simulink model "Full_System_Test"  (R2023a)
settings: Solver=ode23tb  StartTime=0.0  StopTime=3  RelTol=1e-3
libraries: dspfdesign x8, dspsrcs4 x8, dspvision x2, dspxfrm3 x1
settings Model: Creator=zacha  LastModifiedBy=zacha
settings DebuggingCC: UnconnectedInputMsg=warning  UnconnectedOutputMsg=warning  UnconnectedLineMsg=warning
settings ModelReferenceCC: EnableRefExpFcnMdlSchedulingChecks=on
settings RTWCC: DLArmComputeVersion=19.05

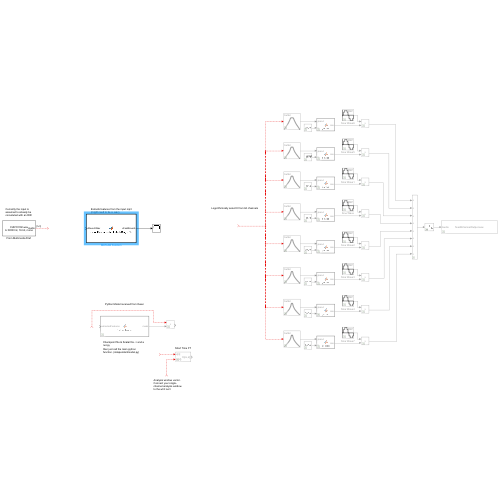
[thumbnail: Simulink's stored preview of the top-level diagram]
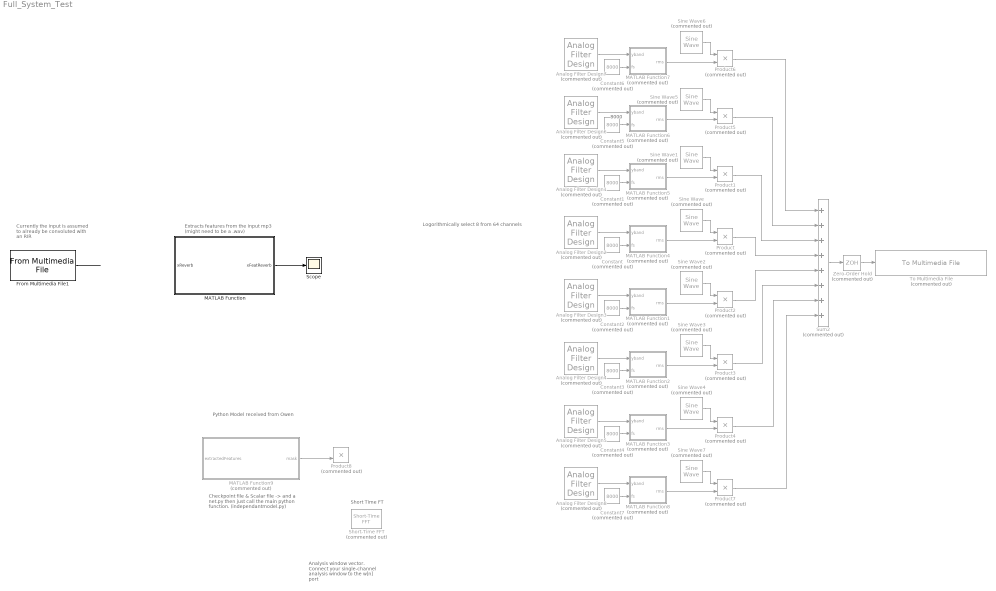
== system Full_System_Test ==
  note: Logorithmically select 8 from 64 channels
  note: Currently the input is assumed to already be convoluted with an RIR
  note: 8000
  note: Short Time FT
  note: Analysis window vector. Connect your single-channel analysis window to the w[n] port
  note: Checkpoint file & Scalar file -> and a net.py
      | then just call the main python function. (independantmodel.py)
  note: Python Model received from Owen
  note: Extracts features from the input mp3 (might need to be a .wav)
  Analog Filter Design1 : dspfdesign/Analog Filter Design  Commented=on  method=Butterworth  filttype=Bandpass  N=6  Wlo=5497.89355477605  Whi=8266.17682725960  Rp=2  Rs=40
  Analog Filter Design2 : dspfdesign/Analog Filter Design  Commented=on  method=Butterworth  filttype=Bandpass  N=6  Wlo=8266.17682725960  Whi=11762.6119981492  Rp=2  Rs=40
  Analog Filter Design3 : dspfdesign/Analog Filter Design  Commented=on  method=Butterworth  filttype=Bandpass  N=6  Wlo=11762.6119981492  Whi=16178.7275834830  Rp=2  Rs=40
  Analog Filter Design4 : dspfdesign/Analog Filter Design  Commented=on  method=Butterworth  filttype=Bandpass  N=6  Wlo=16178.7275834830  Whi=21756.4305609036  Rp=2  Rs=40
  Analog Filter Design5 : dspfdesign/Analog Filter Design  Commented=on  method=Butterworth  filttype=Bandpass  N=6  Wlo=21756.4305609036  Whi=28801.2576047532  Rp=2  Rs=40
  Analog Filter Design6 : dspfdesign/Analog Filter Design  Commented=on  method=Butterworth  filttype=Bandpass  N=6  Wlo=3306.12053392451  Whi=5497.89355477605  Rp=2  Rs=40
  Analog Filter Design7 : dspfdesign/Analog Filter Design  Commented=on  method=Butterworth  filttype=Bandpass  N=6  Wlo=1570.79632679490  Whi=3306.12053392451  Rp=2  Rs=40
  Analog Filter Design8 : dspfdesign/Analog Filter Design  Commented=on  method=Butterworth  filttype=Bandpass  N=6  Wlo=28801.2576047532  Whi=37699.1118430775  Rp=2  Rs=40
  Constant{,1..7} (8 alike) : Constant  Commented=on  Value=8000
  From Multimedia File1 : dspvision/From Multimedia File  inputFilename=C:\Users\zacha\Desktop\Cochlear\Media\zach reverb audio\zach reverb audio\CUNY0102.wav  readRange=[1 Inf]  loop=on  numPlays=1  outputStreams=Audio only  videoDataType=single  audioDataType=double  inheritSampleTime=off  userDefinedSampleTime=1/8000  noAudioOutput=off  isIntensityVideo=off  fourcc=RGB  colorVideoFormat=Separate color signals  outputEOF=off  dataOrg=Column-major  audioFrameSize=1  computeAudioFrameSize=off  outSamplingMode=Sample based
      settings: LibrarySourceBlock=dspsrcs4/From Multimedia File
  MATLAB Function : MATLAB Function  TreatAsAtomicUnit=on
  MATLAB Function1 : MATLAB Function  Commented=on  TreatAsAtomicUnit=on
  MATLAB Function2 : MATLAB Function  Commented=on  TreatAsAtomicUnit=on
  MATLAB Function3 : MATLAB Function  Commented=on  TreatAsAtomicUnit=on
  MATLAB Function4 : MATLAB Function  Commented=on  TreatAsAtomicUnit=on
  MATLAB Function5 : MATLAB Function  Commented=on  TreatAsAtomicUnit=on
  MATLAB Function6 : MATLAB Function  Commented=on  TreatAsAtomicUnit=on
  MATLAB Function7 : MATLAB Function  Commented=on  TreatAsAtomicUnit=on
  MATLAB Function8 : MATLAB Function  Commented=on  TreatAsAtomicUnit=on
  MATLAB Function9 : MATLAB Function  Commented=on  TreatAsAtomicUnit=on
  Product{,1..8} (9 alike) : Product  Commented=on
  Scope : Scope
  Short-Time FFT : dspxfrm3/Short-Time FFT  Commented=on  W=512  OvLap=384  M=1024
  Sine Wave : dspsrcs4/Sine Wave  Commented=on  Amplitude=1  Frequency=1593.84037285376  Phase=0  SampleMode=Discrete  OutComplex=Real  CompMethod=Trigonometric fcn  TableSize=Speed  SampleTime=1/8000  SamplesPerFrame=1  ResetState=Restart at time zero  OutputFrames=off  dataType=double  wordLen=16  udDataType=sfix(16)  fracBitsMode=Best precision  numFracBits=15  OutDataTypeStr=double  LastOutDataTypeStr=double
  Sine Wave1 : dspsrcs4/Sine Wave  Commented=on  Amplitude=1  Frequency=1095.30991918286  Phase=0  SampleMode=Discrete  OutComplex=Real  CompMethod=Trigonometric fcn  TableSize=Speed  SampleTime=1/8000  SamplesPerFrame=1  ResetState=Restart at time zero  OutputFrames=off  dataType=double  wordLen=16  udDataType=sfix(16)  fracBitsMode=Best precision  numFracBits=15  OutDataTypeStr=double  LastOutDataTypeStr=double
  Sine Wave2 : dspsrcs4/Sine Wave  Commented=on  Amplitude=1  Frequency=2223.50115551300  Phase=0  SampleMode=Discrete  OutComplex=Real  CompMethod=Trigonometric fcn  TableSize=Speed  SampleTime=1/8000  SamplesPerFrame=1  ResetState=Restart at time zero  OutputFrames=off  dataType=double  wordLen=16  udDataType=sfix(16)  fracBitsMode=Best precision  numFracBits=15  OutDataTypeStr=double  LastOutDataTypeStr=double
  Sine Wave3 : dspsrcs4/Sine Wave  Commented=on  Amplitude=1  Frequency=3018.78396782595  Phase=0  SampleMode=Discrete  OutComplex=Real  CompMethod=Trigonometric fcn  TableSize=Speed  SampleTime=1/8000  SamplesPerFrame=1  ResetState=Restart at time zero  OutputFrames=off  dataType=double  wordLen=16  udDataType=sfix(16)  fracBitsMode=Best precision  numFracBits=15  OutDataTypeStr=double  LastOutDataTypeStr=double
  Sine Wave4 : dspsrcs4/Sine Wave  Commented=on  Amplitude=1  Frequency=4023.25299143145  Phase=0  SampleMode=Discrete  OutComplex=Real  CompMethod=Trigonometric fcn  TableSize=Speed  SampleTime=1/8000  SamplesPerFrame=1  ResetState=Restart at time zero  OutputFrames=off  dataType=double  wordLen=16  udDataType=sfix(16)  fracBitsMode=Best precision  numFracBits=15  OutDataTypeStr=double  LastOutDataTypeStr=double
  Sine Wave5 : dspsrcs4/Sine Wave  Commented=on  Amplitude=1  Frequency=700.601180633691  Phase=0  SampleMode=Discrete  OutComplex=Real  CompMethod=Trigonometric fcn  TableSize=Speed  SampleTime=1/8000  SamplesPerFrame=1  ResetState=Restart at time zero  OutputFrames=off  dataType=double  wordLen=16  udDataType=sfix(16)  fracBitsMode=Best precision  numFracBits=15  OutDataTypeStr=double  LastOutDataTypeStr=double
  Sine Wave6 : dspsrcs4/Sine Wave  Commented=on  Amplitude=1  Frequency=388.092712715851  Phase=0  SampleMode=Discrete  OutComplex=Real  CompMethod=Trigonometric fcn  TableSize=Speed  SampleTime=1/8000  SamplesPerFrame=1  ResetState=Restart at time zero  OutputFrames=off  dataType=double  wordLen=16  udDataType=sfix(16)  fracBitsMode=Best precision  numFracBits=15  OutDataTypeStr=double  LastOutDataTypeStr=double
  Sine Wave7 : dspsrcs4/Sine Wave  Commented=on  Amplitude=1  Frequency=5291.93125752976  Phase=0  SampleMode=Discrete  OutComplex=Real  CompMethod=Trigonometric fcn  TableSize=Speed  SampleTime=1/8000  SamplesPerFrame=1  ResetState=Restart at time zero  OutputFrames=off  dataType=double  wordLen=16  udDataType=sfix(16)  fracBitsMode=Best precision  numFracBits=15  OutDataTypeStr=double  LastOutDataTypeStr=double
  Sum2 : Sum  Commented=on  Inputs=++++++++
  To Multimedia File : dspvision/To Multimedia File  Commented=on  outputFilename=C:\Users\zacha\Desktop\Cochlear\Media\fixed8channelOutput.wav  streamSelection=Audio only  videoCompressor=None (uncompressed)  audioCompressor=None (uncompressed)  imagePorts=Separate color signals  fileType=WAV  audioDatatype=16-bit integer  fourcc=RGB  videoQuality=75  mj2000CompFactor=10
      settings: LibrarySourceBlock=dspsnks4/To Multimedia File
  Zero-Order Hold : ZeroOrderHold  Commented=on  SampleTime=-1
  wires:
  Analog Filter Design2/1 -> MATLAB Function4/1(yband)
  Constant/1 -> MATLAB Function4/2(fs)
  MATLAB Function4/1(rms) -> Product/2
  Sine Wave/1 -> Product/1
  Sine Wave1/1 -> Product1/1
  Analog Filter Design1/1 -> MATLAB Function5/1(yband)
  MATLAB Function5/1(rms) -> Product1/2
  Constant1/1 -> MATLAB Function5/2(fs)
  Sine Wave2/1 -> Product2/1
  Analog Filter Design3/1 -> MATLAB Function1/1(yband)
  MATLAB Function1/1(rms) -> Product2/2
  Constant2/1 -> MATLAB Function1/2(fs)
  Sine Wave3/1 -> Product3/1
  MATLAB Function2/1(rms) -> Product3/2
  Analog Filter Design4/1 -> MATLAB Function2/1(yband)
  Constant3/1 -> MATLAB Function2/2(fs)
  Sine Wave4/1 -> Product4/1
  MATLAB Function3/1(rms) -> Product4/2
  Analog Filter Design5/1 -> MATLAB Function3/1(yband)
  Constant4/1 -> MATLAB Function3/2(fs)
  Sine Wave5/1 -> Product5/1
  MATLAB Function6/1(rms) -> Product5/2
  Analog Filter Design6/1 -> MATLAB Function6/1(yband)
  Constant5/1 -> MATLAB Function6/2(fs)
  Product/1 -> Sum2/4
  Product2/1 -> Sum2/5
  Product1/1 -> Sum2/3
  Product5/1 -> Sum2/2
  Product3/1 -> Sum2/6
  Product4/1 -> Sum2/7
  Zero-Order Hold/1 -> To Multimedia File/1
  Sum2/1 -> Zero-Order Hold/1
  Constant6/1 -> MATLAB Function7/2(fs)
  MATLAB Function7/1(rms) -> Product6/2
  Analog Filter Design7/1 -> MATLAB Function7/1(yband)
  Sine Wave6/1 -> Product6/1
  Product6/1 -> Sum2/1
  Constant7/1 -> MATLAB Function8/2(fs)
  MATLAB Function8/1(rms) -> Product7/2
  ? -> Analog Filter Design7/1, Analog Filter Design6/1, Analog Filter Design1/1, Analog Filter Design2/1, Analog Filter Design8/1, Analog Filter Design5/1, Analog Filter Design4/1, Analog Filter Design3/1
  Analog Filter Design8/1 -> MATLAB Function8/1(yband)
  Sine Wave7/1 -> Product7/1
  Product7/1 -> Sum2/8
  From Multimedia File1/1 -> ?
  ? -> Short-Time FFT/1
  ? -> Short-Time FFT/2
  MATLAB Function9/1(mask) -> Product8/2
  ? -> Product8/1
  MATLAB Function/1(xFeatReverb) -> Scope/1

== matlab function Full_System_Test/MATLAB Function2 ==
  data: yband input; rms output; fs input
function rms = getrms(yband,fs)

    y = abs(yband); %rectifying it makes it sound bad

    [b,a] = butter(2,400/(fs/2));

    z = filter(b,a,y); %this filter also makes it sound bad

    windowsize = round(4/(1000/fs)); %rms computed every 4ms = windowsize samples

    [yupper,ylower] = envelope(yband,windowsize,'rms'); %changed to yband here

    %envelope(z,windowsize,'rms');

    rms = yupper;
end

== matlab function Full_System_Test/MATLAB Function3 ==
  data: yband input; rms output; fs input
function rms = getrms(yband,fs)

    y = abs(yband); %rectifying it makes it sound bad

    [b,a] = butter(2,400/(fs/2));

    z = filter(b,a,y); %this filter also makes it sound bad

    windowsize = round(4/(1000/fs)); %rms computed every 4ms = windowsize samples

    [yupper,ylower] = envelope(yband,windowsize,'rms'); %changed to yband here

    %envelope(z,windowsize,'rms');

    rms = yupper;
end

== matlab function Full_System_Test/MATLAB Function6 ==
  data: yband input; rms output; fs input
function rms = getrms(yband,fs)

    y = abs(yband); %rectifying it makes it sound bad

    [b,a] = butter(2,400/(fs/2));

    z = filter(b,a,y); %this filter also makes it sound bad

    windowsize = round(4/(1000/fs)); %rms computed every 4ms = windowsize samples

    [yupper,ylower] = envelope(yband,windowsize,'rms'); %changed to yband here

    %envelope(z,windowsize,'rms');

    rms = yupper;
end

== matlab function Full_System_Test/MATLAB Function4 ==
  data: yband input; rms output; fs input
function rms = getrms(yband,fs)

    y = abs(yband); %rectifying it makes it sound bad

    [b,a] = butter(2,400/(fs/2));

    z = filter(b,a,y); %this filter also makes it sound bad

    windowsize = round(4/(1000/fs)); %rms computed every 4ms = windowsize samples

    [yupper,ylower] = envelope(yband,windowsize,'rms'); %changed to yband here

    %envelope(z,windowsize,'rms');

    rms = yupper;
end

== matlab function Full_System_Test/MATLAB Function5 ==
  data: yband input; rms output; fs input
function rms = getrms(yband,fs)

    y = abs(yband); %rectifying it makes it sound bad

    [b,a] = butter(2,400/(fs/2));

    z = filter(b,a,y); %this filter also makes it sound bad

    windowsize = round(4/(1000/fs)); %rms computed every 4ms = windowsize samples

    [yupper,ylower] = envelope(yband,windowsize,'rms'); %changed to yband here

    %envelope(z,windowsize,'rms');

    rms = yupper;
end

== matlab function Full_System_Test/MATLAB Function7 ==
  data: yband input; rms output; fs input
function rms = getrms(yband,fs)

    y = abs(yband); %rectifying it makes it sound bad

    [b,a] = butter(2,400/(fs/2));

    z = filter(b,a,y); %this filter also makes it sound bad

    windowsize = round(4/(1000/fs)); %rms computed every 4ms = windowsize samples

    [yupper,ylower] = envelope(yband,windowsize,'rms'); %changed to yband here

    %envelope(z,windowsize,'rms');

    rms = yupper;
end

== matlab function Full_System_Test/MATLAB Function8 ==
  data: yband input; rms output; fs input
function rms = getrms(yband,fs)

    y = abs(yband); %rectifying it makes it sound bad

    [b,a] = butter(2,400/(fs/2));

    z = filter(b,a,y); %this filter also makes it sound bad

    windowsize = round(4/(1000/fs)); %rms computed every 4ms = windowsize samples

    [yupper,ylower] = envelope(yband,windowsize,'rms'); %changed to yband here

    %envelope(z,windowsize,'rms');

    rms = yupper;
end

== matlab function Full_System_Test/MATLAB Function ==
  data: xReverb input; xFeatReverb output
%[xAnechoic,fs] = audioread(wavFile); % change this to read in your mp3

% you can use simulink to get the reverb from the xAnechoic
% xReverb = [1,2,3,4] % this is where you can put in your reverberant signal for now

%xFeatReverb = extractFeaturesAndLabelsSingleFile(xReverb)


function xFeatReverb = extractFeaturesAndLabelsSingleFile(xReverb)
    % Feature extraction/mask calculation parameters
    feat_type = 'log_fft_889Hz_preemph';
    fs = 8000; % Hz
    frame_len = 0.008; % s
    %frame_shift = 0.002; % s
    frame_shift = 9/8000; % based on channel stimulation rate from clinical map, seconds
    preemphasis = true;

    %[xReverb,~] = audioread(xReverbWav); 
    
    %
    % OLD Args:
    %   -wavFile (str): .wav file from which to extract features
    %   -feat_type (str): feature type (mfcc or log mel spectrogram)
    %   -mask_type (str): binary, ratio, or fft mask
    %   -ftm_type_mask (str): frequency-time representation to use for mask
    %   calculation (FFT or ACE magnitude spectrum)
    %   -fs (double): sampling frequency in Hz
    %   -frame_len (double): FFT frame length in sec
    %   -frame_shift (double): FFT frame shift in sec
    %   -num_coeffs (int): dimensionality of feature vector at single time step
    %   -preemphasis (bool): whether to apply pre-emphasis filter
    %   -use_energy (bool): whether to use energy as an additional feature
    %   -featFile (str): file containing extracted features and labels
    %   -rir_file (str): name of file that contains the RIR, could be either
    %   a .mat file or a .wav file
    %   -rir_database (str): name of RIR database
    %   -corpus (str): name of speech corpus
    %   -ali_contents (str): contents of the phoneme alignment file
    %
    

    % Apply pre-emphasis, if desired
    if preemphasis
      xReverb = preemphasize(xReverb);

      % Re-normalize
      normFactor = 0.99/max(abs(xReverb));
      xReverb = xReverb*normFactor;
    end
    
    % Extract features
    xFeatReverb = extractFeatures(xReverb, feat_type, fs, frame_len, frame_shift);
    
end

function x = extractFeatures(wav, feat_type, fs, frame_len, frame_shift)
    % Calculate static features for a single wav file
    %
    % Args:
    %   -wav (nx1 array): audio data
    %   -feat_type (str): name of feature
    %   -fs (double): sampling frequency in Hz
    %   -frame_len (double): FFT frame length, sec
    %   -frame_shift (double): FFT frame shift, sec
    %
    % Returns:
    %   -x (nxnFeatures matrix): matrix of features

  % Default ACE map in Nucleus MATLAB Toolbox
  p = ACE_map;

  % Replace default block length and analysis rate with user-defined parameters
  p.block_length = round(frame_len*fs);
  p.analysis_rate = 1/frame_shift;

    % Calculate either mel-frequency cepstral coefficients (mfcc) or log
    % mel spectrogram (mspec)
    switch feat_type
        % ACE power spectrum
        case 'ace'
	    x = calculateAceFeatures(p, wav);

        % log ACE power spectrum
        case 'log_ace'
	    x = calculateAceFeatures(p, wav);
	    x = log(x);
            
        % log FFT power spectrum
        case 'log_fft'
	    x = calculateFftFeatures(p, wav);
	    x = log(x);
            
        otherwise
	    if contains(feat_type, 'log_fft')
	        x = calculateFftFeatures(p, wav);
	        x = log(x);
	    else
              error('Invalid feature type.\n');
	    end
    end
    
end

== matlab function Full_System_Test/MATLAB Function9 ==
  data: extractedFeatures input; mask output
function mask = PythonModel(extractedFeatures)
    mask = 0; % Has to be preassigned, otherwise Simulink throws an error
    coder.extrinsic('py.models.test') % Python functions have to be run extrinsically, meaning no C code generated
    mask = py.models.test(extractedFeatures);
end

== matlab function Full_System_Test/MATLAB Function1 ==
  data: yband input; rms output; fs input
function rms = getrms(yband,fs)

    y = abs(yband); %rectifying it makes it sound bad

    [b,a] = butter(2,400/(fs/2));

    z = filter(b,a,y); %this filter also makes it sound bad

    windowsize = round(4/(1000/fs)); %rms computed every 4ms = windowsize samples

    [yupper,ylower] = envelope(yband,windowsize,'rms'); %changed to yband here

    %envelope(z,windowsize,'rms');

    rms = yupper;
end
